simulink model "PID_Controller"  (R2024b)
settings: Solver=VariableStepAuto  StartTime=0.0  StopTime=10.0  RelTol=1e-3
undefined symbols (not defined in the file): gravity, initial_altitide, initial_velocity, mass
settings Model: Creator=Metabox  LastModifiedBy=Metabox

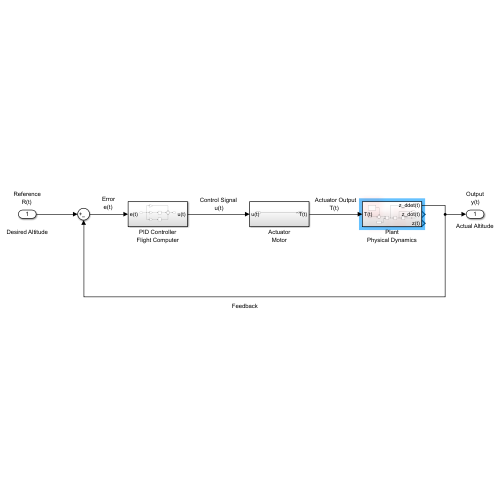
[thumbnail: Simulink's stored preview of the top-level diagram]
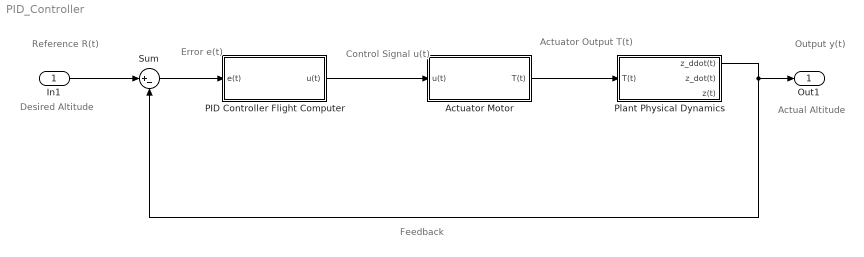
== system PID_Controller ==
  note: Reference
      |      R(t)
  note: Output
      |    y(t)
  note: Feedback
  note: Error
      |  e(t)
  note: Control Signal
      |          u(t)
  note: Actuator Output
      |          T(t)
  note: Actual Altitude
  note: Desired Altitude
  In1 : Inport
  Actuator Motor : Subsystem
  PID Controller Flight Computer : Subsystem
  Plant Physical Dynamics : Subsystem
  Sum : Sum  Inputs=|+-
  Out1 : Outport
  wires:
  In1/1 -> Sum/1
  Sum/1 -> PID Controller Flight Computer/1(e(t))
  PID Controller Flight Computer/1(u(t)) -> Actuator Motor/1(u(t))
  Actuator Motor/1(T(t)) -> Plant Physical Dynamics/1(T(t))
  Plant Physical Dynamics/1(z_ddot(t)) -> Sum/2, Out1/1

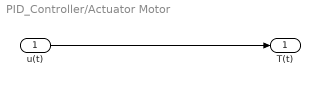
== system PID_Controller/Actuator Motor ==
  u(t) : Inport
  T(t) : Outport
  wires:
  u(t)/1 -> T(t)/1

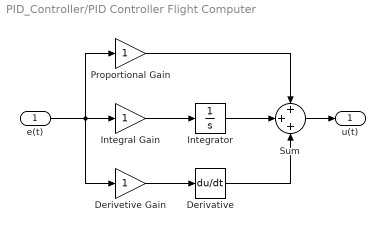
== system PID_Controller/PID Controller Flight Computer ==
  e(t) : Inport
  Derivative : Derivative
  Derivetive Gain : Gain
  Integral Gain : Gain
  Integrator : Integrator
      settings: AttributesFormatString=Integrator
  Proportional Gain : Gain
  Sum : Sum  Inputs=+++
  u(t) : Outport
  wires:
  e(t)/1 -> Derivetive Gain/1, Proportional Gain/1, Integral Gain/1
  Integral Gain/1 -> Integrator/1
  Integrator/1 -> Sum/2
  Derivetive Gain/1 -> Derivative/1
  Derivative/1 -> Sum/3
  Proportional Gain/1 -> Sum/1
  Sum/1 -> u(t)/1

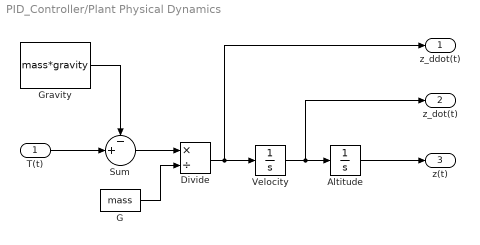
== system PID_Controller/Plant Physical Dynamics ==
  T(t) : Inport
  Altitude : Integrator  InitialCondition=initial_altitide  ContinuousStateAttributes=altitude
  Divide : Product  Inputs=*/
  G : Constant  Value=mass
  Gravity : Constant  Value=mass*gravity
  Sum : Sum  Inputs=-+|
  Velocity : Integrator  InitialCondition=initial_velocity  ContinuousStateAttributes=velocity
  z_ddot(t) : Outport
  z_dot(t) : Outport  Port=2
  z(t) : Outport  Port=3
  wires:
  T(t)/1 -> Sum/2
  Velocity/1 -> z_dot(t)/1, Altitude/1
  Altitude/1 -> z(t)/1
  Divide/1 -> z_ddot(t)/1, Velocity/1
  Sum/1 -> Divide/1
  Gravity/1 -> Sum/1
  G/1 -> Divide/2
